simulink model "EPT"  (R2019b)
settings: Solver=FixedStepDiscrete  StartTime=0.0  StopTime=5  FixedStep=0.005  RelTol=1e-3  EnableMultiTasking=on
PreLoadFcn:
  | try, model_open; catch, disp('Error occurred while executing model pre-load callback: model_open.m'); disp('Please assure that the MATLAB working directory is set to the model directory before opening.'); end
InitFcn:
  | try, model_open; catch, end
undefined symbols (not defined in the file or in its folder): Bridge, GCM, H, ln, raptor_get_param_eval, raptor_get_safe_string, raptor_xcp_function
libraries: Raptor_lib x2810, simulink x374, hdlsllib x19
(part 12 of 45)

== system EPT/Foreground_TimeBase_5ms/CAN/CAN1_exec/BCU vs RMDA-BMS/BCU-OBU Status-OP G2 ==
  Trigger : TriggerPort  VariantControl=Variant  PortDimensions=1
  raptor_adjustment : Raptor_lib/Data Storage/raptor_adjustment  paramName='Cal_BP_OBU_AH_Def'  nameSource=Parameter  initValue=145  dataType=uint8  storage=Calibration  calDispType=Number  calEnum={'False', 'True'}  calGain=1.0  calOffset=0.0  calMax=inf  calMin=-inf  calFormat='-1'  calUnit=''  calHelp=''  calAccess=1  calFunction=raptor_xcp_function(gcb)  calDispHeaders=off  calColHeaders={'Col1' 'Col2' 'Col3'}  calRowHeaders={'Row1' 'Row2' 'Row3'}
      settings: SourceProductName=Raptor
  raptor_can_txmsg : Raptor_lib/CAN/raptor_can_txmsg  canDefinition=struct('dbcFile', 'BCU_OBU_HMI.dbc','message', 'BCU_OBU_Status_OP_G2','comment', '','signals', {{'BP_OBU_SOA','BP_OBU_SOC','BP_OBU_AH_Stored','BP_OBU_AH_FCC','BP_OBU_AH_Def'}},'enabled', [ 1 1 1 1 1;],'canBus', '''CAN1''','messageID', [ 1526;],'idMask', [ 536870911;],'payloadMask', [],'payloadValue', [],'period', [ 0;],'mailbox', '','queueSize', [ 1;],'label', [ 0;],'ver', [ 2;],'showID', [ 0;],'showRaw', [ 0;],'fill', [ 0;],'editID', [ 0;],'signalOrder', [ 2;])  canBus='CAN1'  queueSize=1  payloadMask=[]  payloadValue=[]  period=0  showID=0  label=0  idMask=hex2dec('1FFFFFFF')  fill=0  id=1526  showRaw=0  signalOrder=2  signalInfo={{struct('Name', 'BP_OBU_AH_Def','Startbit', [ 0;],'SignalSize', [ 8;],'ByteOrder', 'BigEndian','ValueType', 'UNSIGNED','Class', 'uint8','Signed', [ 0;],'Factor', [ 1;],'Offset', [ 0;],'Min', [ 0;],'Max', [ 0;],'Units', '','Comment', '','StartBit', [ 0;]),struct('Name', 'BP_OBU_AH_FCC','Startbit', [ 0;],'SignalSize', [ 8;],'ByteOrder', 'BigEndian','ValueType', 'UNSIGNED','Class', 'uint8','Signed', [ 0;],'Factor', [ 1;],'Offset', [ 0;],'Min', [ 0;],'Max', [ 0;],'Units', '','Comment', '','StartBit', [ 8;]),struct('Name', 'BP_OBU_AH_Stored','Startbit', [ 0;],'SignalSize', [ 8;],'ByteOrder', 'BigEndian','ValueType', 'UNSIGNED','Class', 'uint8','Signed', [ 0;],'Factor', [ 1;],'Offset', [ 0;],'Min', [ 0;],'Max', [ 0;],'Units', '','Comment', '','StartBit', [ 16;]),struct('Name', 'BP_OBU_SOC','Startbit', [ 0;],'SignalSize', [ 16;],'ByteOrder', 'BigEndian','ValueType', 'UNSIGNED','Class', 'uint16','Signed', [ 0;],'Factor', [ 0.1;],'Offset', [ -50;],'Min', [ 0;],'Max', [ 0;],'Units', '','Comment', '','StartBit', [ 32;]),struct('Name', 'BP_OBU_SOA','Startbit', [ 0;],'SignalSize', [ 8;],'ByteOrder', 'BigEndian','ValueType', 'UNSIGNED','Class', 'uint8','Signed', [ 0;],'Factor', [ 0.5;],'Offset', [ 0;],'Min', [ 0;],'Max', [ 0;],'Units', '','Comment', '','StartBit', [ 40;])}}
      settings: SourceProductName=Raptor
  raptor_data_def1 : Raptor_lib/Data Storage/raptor_data_def  dataName='EPT_BPOBU_FCCAP'  initValue=0  dataType=double  storage=Volatile (RAM)  calVisible=on  calType=Measurement  calDispType=Number  calEnum={'False', 'True'}  calGain=1.0  calOffset=0  calMin=-inf  calMax=inf  calFormat='-1'  calUnit=''  calHelp=''  calAccess=1  calFunction=raptor_xcp_function(gcb)  calDispHeaders=off  calColHeaders={'Col1' 'Col2' 'Col3'}  calRowHeaders={'Row1' 'Row2' 'Row3'}
      settings: SourceProductName=Raptor
  raptor_data_def2 : Raptor_lib/Data Storage/raptor_data_def  dataName='EPT_BPOBU_AH_Def'  initValue=0  dataType=uint8  storage=Volatile (RAM)  calVisible=on  calType=Measurement  calDispType=Number  calEnum={'False', 'True'}  calGain=1.0  calOffset=0  calMin=-inf  calMax=inf  calFormat='-1'  calUnit=''  calHelp=''  calAccess=1  calFunction=raptor_xcp_function(gcb)  calDispHeaders=off  calColHeaders={'Col1' 'Col2' 'Col3'}  calRowHeaders={'Row1' 'Row2' 'Row3'}
      settings: SourceProductName=Raptor
  raptor_data_def4 : Raptor_lib/Data Storage/raptor_data_def  dataName='BP_OBU_AH_Stored'  initValue=0  dataType=double  storage=Volatile (RAM)  calVisible=on  calType=Measurement  calDispType=Number  calEnum={'False', 'True'}  calGain=1.0  calOffset=0  calMin=-inf  calMax=inf  calFormat='-1'  calUnit=''  calHelp=''  calAccess=1  calFunction=raptor_xcp_function(gcb)  calDispHeaders=off  calColHeaders={'Col1' 'Col2' 'Col3'}  calRowHeaders={'Row1' 'Row2' 'Row3'}
      settings: SourceProductName=Raptor
  raptor_data_def5 : Raptor_lib/Data Storage/raptor_data_def  dataName='EPT_BPOBU_SOA'  initValue=0  dataType=double  storage=Volatile (RAM)  calVisible=on  calType=Measurement  calDispType=Number  calEnum={'False', 'True'}  calGain=1.0  calOffset=0  calMin=-inf  calMax=inf  calFormat='-1'  calUnit=''  calHelp=''  calAccess=1  calFunction=raptor_xcp_function(gcb)  calDispHeaders=off  calColHeaders={'Col1' 'Col2' 'Col3'}  calRowHeaders={'Row1' 'Row2' 'Row3'}
      settings: SourceProductName=Raptor
  raptor_data_read1 : Raptor_lib/Data Storage/raptor_data_read  dataName='EPT_BPOBU_SOC'  dataShape=Scalar  idxSource=Input  idxRow=1  idxCol=1
      settings: SourceProductName=Raptor
  raptor_data_read2 : Raptor_lib/Data Storage/raptor_data_read  dataName='BP_OBU_AH_Stored'  dataShape=Scalar  idxSource=Input  idxRow=1  idxCol=1
      settings: SourceProductName=Raptor
  raptor_data_read4 : Raptor_lib/Data Storage/raptor_data_read  dataName='EPT_BPOBU_FCCAP'  dataShape=Scalar  idxSource=Input  idxRow=1  idxCol=1
      settings: SourceProductName=Raptor
  raptor_data_read5 : Raptor_lib/Data Storage/raptor_data_read  dataName='EPT_BPOBU_AH_DEF'  dataShape=Scalar  idxSource=Input  idxRow=1  idxCol=1
      settings: SourceProductName=Raptor
  raptor_data_read7 : Raptor_lib/Data Storage/raptor_data_read  dataName='EPT_BPOBU_SOA'  dataShape=Scalar  idxSource=Input  idxRow=1  idxCol=1
      settings: SourceProductName=Raptor
  raptor_data_write : Raptor_lib/Data Storage/raptor_data_write  dataName='EPT_BPOBU_AH_DEF'  dataShape=Scalar  idxSource=Input Port  idxRow=1  idxCol=1
      settings: SourceProductName=Raptor
  wires:
  raptor_data_read5/1 -> raptor_can_txmsg/5
  raptor_data_read4/1 -> raptor_can_txmsg/4
  raptor_data_read1/1 -> raptor_can_txmsg/2
  raptor_data_read2/1 -> raptor_can_txmsg/3
  raptor_data_read7/1 -> raptor_can_txmsg/1
  raptor_adjustment/1 -> raptor_data_write/1

== system EPT/Foreground_TimeBase_5ms/CAN/CAN1_exec/BCU vs RMDA-BMS/BCU-OBU Status-OP G3 ==
  Trigger : TriggerPort  VariantControl=Variant  PortDimensions=1
  raptor_can_txmsg : Raptor_lib/CAN/raptor_can_txmsg  canDefinition=struct('dbcFile', 'BCU_OBU_HMI.dbc','message', 'BCU_OBU_Status_OP_G3','comment', '','signals', {{'NA_Cooling_CTL_OP','I2V_Batt_Volt','BP_OBU_Tair_in','BP_OBU_Tair_Out','BP_OBU_Tbp_Down','BP_OBU_Tbp_Up'}},'enabled', [ 1 1 1 1 1 1;],'canBus', '''CAN1''','messageID', [ 1527;],'idMask', [ 536870911;],'payloadMask', [],'payloadValue', [],'period', [ 0;],'mailbox', '','queueSize', [ 1;],'label', [ 0;],'ver', [ 2;],'showID', [ 0;],'showRaw', [ 0;],'fill', [ 0;],'editID', [ 0;],'signalOrder', [ 2;])  canBus='CAN1'  queueSize=1  payloadMask=[]  payloadValue=[]  period=0  showID=0  label=0  idMask=hex2dec('1FFFFFFF')  fill=0  id=1527  showRaw=0  signalOrder=2  signalInfo={{struct('Name', 'BP_OBU_Tbp_Up','Startbit', [ 0;],'SignalSize', [ 8;],'ByteOrder', 'BigEndian','ValueType', 'UNSIGNED','Class', 'uint8','Signed', [ 0;],'Factor', [ 0.5;],'Offset', [ -40;],'Min', [ 0;],'Max', [ 0;],'Units', '','Comment', '','StartBit', [ 0;]),struct('Name', 'BP_OBU_Tbp_Down','Startbit', [ 0;],'SignalSize', [ 8;],'ByteOrder', 'BigEndian','ValueType', 'UNSIGNED','Class', 'uint8','Signed', [ 0;],'Factor', [ 0.5;],'Offset', [ -40;],'Min', [ 0;],'Max', [ 0;],'Units', '','Comment', '','StartBit', [ 8;]),struct('Name', 'BP_OBU_Tair_Out','Startbit', [ 0;],'SignalSize', [ 8;],'ByteOrder', 'BigEndian','ValueType', 'UNSIGNED','Class', 'uint8','Signed', [ 0;],'Factor', [ 0.5;],'Offset', [ -40;],'Min', [ 0;],'Max', [ 0;],'Units', '','Comment', '','StartBit', [ 16;]),struct('Name', 'BP_OBU_Tair_in','Startbit', [ 0;],'SignalSize', [ 8;],'ByteOrder', 'BigEndian','ValueType', 'UNSIGNED','Class', 'uint8','Signed', [ 0;],'Factor', [ 0.5;],'Offset', [ -40;],'Min', [ 0;],'Max', [ 0;],'Units', '','Comment', '','StartBit', [ 24;]),struct('Name', 'I2V_Batt_Volt','Startbit', [ 0;],'SignalSize', [ 8;],'ByteOrder', 'BigEndian','ValueType', 'UNSIGNED','Class', 'uint8','Signed', [ 0;],'Factor', [ 0.1;],'Offset', [ 0;],'Min', [ 0;],'Max', [ 0;],'Units', '','Comment', '','StartBit', [ 32;]),struct('Name', 'NA_Cooling_CTL_OP','Startbit', [ 0;],'SignalSize', [ 8;],'ByteOrder', 'BigEndian','ValueType', 'UNSIGNED','Class', 'uint8','Signed', [ 0;],'Factor', [ 0.5;],'Offset', [ 0;],'Min', [ 0;],'Max', [ 0;],'Units', '','Comment', '','StartBit', [ 40;])}}
      settings: SourceProductName=Raptor
  raptor_data_def1 : Raptor_lib/Data Storage/raptor_data_def  dataName='BP_OBU_Tair_In'  initValue=0  dataType=double  storage=Volatile (RAM)  calVisible=on  calType=Measurement  calDispType=Number  calEnum={'False', 'True'}  calGain=1.0  calOffset=0  calMin=-inf  calMax=inf  calFormat='-1'  calUnit=''  calHelp=''  calAccess=1  calFunction=raptor_xcp_function(gcb)  calDispHeaders=off  calColHeaders={'Col1' 'Col2' 'Col3'}  calRowHeaders={'Row1' 'Row2' 'Row3'}
      settings: SourceProductName=Raptor
  raptor_data_def2 : Raptor_lib/Data Storage/raptor_data_def  dataName='BP_OBU_Tair_Out'  initValue=0  dataType=double  storage=Volatile (RAM)  calVisible=on  calType=Measurement  calDispType=Number  calEnum={'False', 'True'}  calGain=1.0  calOffset=0  calMin=-inf  calMax=inf  calFormat='-1'  calUnit=''  calHelp=''  calAccess=1  calFunction=raptor_xcp_function(gcb)  calDispHeaders=off  calColHeaders={'Col1' 'Col2' 'Col3'}  calRowHeaders={'Row1' 'Row2' 'Row3'}
      settings: SourceProductName=Raptor
  raptor_data_read1 : Raptor_lib/Data Storage/raptor_data_read  dataName='I2V_Battery_Volt'  dataShape=Scalar  idxSource=Input  idxRow=1  idxCol=1
      settings: SourceProductName=Raptor
  raptor_data_read3 : Raptor_lib/Data Storage/raptor_data_read  dataName='BP_OBU_Tair_In'  dataShape=Scalar  idxSource=Input  idxRow=1  idxCol=1
      settings: SourceProductName=Raptor
  raptor_data_read4 : Raptor_lib/Data Storage/raptor_data_read  dataName='BP_OBU_Tair_Out'  dataShape=Scalar  idxSource=Input  idxRow=1  idxCol=1
      settings: SourceProductName=Raptor
  raptor_data_read5 : Raptor_lib/Data Storage/raptor_data_read  dataName='BP_OBU_Tbp_Down'  dataShape=Scalar  idxSource=Input  idxRow=1  idxCol=1
      settings: SourceProductName=Raptor
  raptor_data_read6 : Raptor_lib/Data Storage/raptor_data_read  dataName='BP_OBU_Tbp_Up'  dataShape=Scalar  idxSource=Input  idxRow=1  idxCol=1
      settings: SourceProductName=Raptor
  wires:
  raptor_data_read1/1 -> raptor_can_txmsg/2
  raptor_data_read4/1 -> raptor_can_txmsg/4
  raptor_data_read5/1 -> raptor_can_txmsg/5
  raptor_data_read6/1 -> raptor_can_txmsg/6
  raptor_data_read3/1 -> raptor_can_txmsg/3

== system EPT/Foreground_TimeBase_5ms/CAN/CAN1_exec/BCU vs RMDA-BMS/BCU-OBU Status-OP G4  ==
  Trigger : TriggerPort  VariantControl=Variant  PortDimensions=1
  raptor_can_txmsg : Raptor_lib/CAN/raptor_can_txmsg  canDefinition=struct('dbcFile', 'BCU_OBU_HMI.dbc','message', 'BCU_OBU_Status_OP_G4','comment', '','signals', {{'Min_CellT','Max_CellT','Min_CellV','Max_CellV'}},'enabled', [ 1 1 1 1;],'canBus', '''CAN1''','messageID', [ 1528;],'idMask', [ 536870911;],'payloadMask', [],'payloadValue', [],'period', [ 0;],'mailbox', '','queueSize', [ 1;],'label', [ 0;],'ver', [ 2;],'showID', [ 0;],'showRaw', [ 0;],'fill', [ 0;],'editID', [ 0;],'signalOrder', [ 2;])  canBus='CAN1'  queueSize=1  payloadMask=[]  payloadValue=[]  period=0  showID=0  label=0  idMask=hex2dec('1FFFFFFF')  fill=0  id=1528  showRaw=0  signalOrder=2  signalInfo={{struct('Name', 'Max_CellV','Startbit', [ 0;],'SignalSize', [ 16;],'ByteOrder', 'BigEndian','ValueType', 'UNSIGNED','Class', 'uint16','Signed', [ 0;],'Factor', [ 0.001;],'Offset', [ 0;],'Min', [ 0;],'Max', [ 0;],'Units', '','Comment', '','StartBit', [ 8;]),struct('Name', 'Min_CellV','Startbit', [ 0;],'SignalSize', [ 16;],'ByteOrder', 'BigEndian','ValueType', 'UNSIGNED','Class', 'uint16','Signed', [ 0;],'Factor', [ 0.001;],'Offset', [ 0;],'Min', [ 0;],'Max', [ 0;],'Units', '','Comment', '','StartBit', [ 24;]),struct('Name', 'Max_CellT','Startbit', [ 0;],'SignalSize', [ 8;],'ByteOrder', 'BigEndian','ValueType', 'UNSIGNED','Class', 'uint8','Signed', [ 0;],'Factor', [ 0.5;],'Offset', [ -40;],'Min', [ 0;],'Max', [ 0;],'Units', '','Comment', '','StartBit', [ 32;]),struct('Name', 'Min_CellT','Startbit', [ 0;],'SignalSize', [ 8;],'ByteOrder', 'BigEndian','ValueType', 'UNSIGNED','Class', 'uint8','Signed', [ 0;],'Factor', [ 0.5;],'Offset', [ -40;],'Min', [ 0;],'Max', [ 0;],'Units', '','Comment', '','StartBit', [ 40;])}}
      settings: SourceProductName=Raptor
  raptor_data_read1 : Raptor_lib/Data Storage/raptor_data_read  dataName='Max_CellT'  dataShape=Scalar  idxSource=Input  idxRow=1  idxCol=1
      settings: SourceProductName=Raptor
  raptor_data_read2 : Raptor_lib/Data Storage/raptor_data_read  dataName='Min_CellT'  dataShape=Scalar  idxSource=Input  idxRow=1  idxCol=1
      settings: SourceProductName=Raptor
  raptor_data_read4 : Raptor_lib/Data Storage/raptor_data_read  dataName='Max_CellV'  dataShape=Scalar  idxSource=Input  idxRow=1  idxCol=1
      settings: SourceProductName=Raptor
  raptor_data_read5 : Raptor_lib/Data Storage/raptor_data_read  dataName='Min_CellV'  dataShape=Scalar  idxSource=Input  idxRow=1  idxCol=1
      settings: SourceProductName=Raptor
  wires:
  raptor_data_read5/1 -> raptor_can_txmsg/3
  raptor_data_read4/1 -> raptor_can_txmsg/4
  raptor_data_read1/1 -> raptor_can_txmsg/2
  raptor_data_read2/1 -> raptor_can_txmsg/1

== system EPT/Foreground_TimeBase_5ms/CAN/CAN1_exec/BCU vs RMDA-BMS/BP-OBU Enable CTL & OP Status  ==
  Trigger : TriggerPort  VariantControl=Variant  PortDimensions=1
  BP-OBU Enable CTL : Subsystem
  BP-OBU Output Mode : Subsystem
  BP-OBU_Enable Mode : Subsystem
  BP-OBU_HV CTL Mode : Subsystem
  BP-OBU_OP Mode : Subsystem
  EPT Status Bitmap : Subsystem
  raptor_can_txmsg : Raptor_lib/CAN/raptor_can_txmsg  canDefinition=struct('dbcFile', 'BCU_OBU_HMI.dbc','message', 'BP_OBU_Enable_CTLandOP_Status','comment', '','signals', {{'BP_OBU_HV_CTL_Mode','BP_OBU_Enable_Mode','BP_OBU_OP_Mode','BP_OBU_Output_Mode','BP_OBU_Enable_CTL','EPT_Status_Bitmap'}},'enabled', [ 1 1 1 1 1 1;],'canBus', '''CAN1''','messageID', [ 1523;],'idMask', [ 536870911;],'payloadMask', [],'payloadValue', [],'period', [ 0;],'mailbox', '','queueSize', [ 1;],'label', [ 0;],'ver', [ 2;],'showID', [ 0;],'showRaw', [ 0;],'fill', [ 0;],'editID', [ 0;],'signalOrder', [ 2;])  canBus='CAN1'  queueSize=1  payloadMask=[]  payloadValue=[]  period=0  showID=0  label=0  idMask=hex2dec('1FFFFFFF')  fill=0  id=1523  showRaw=0  signalOrder=2  signalInfo={{struct('Name', 'EPT_Status_Bitmap','Startbit', [ 0;],'SignalSize', [ 8;],'ByteOrder', 'BigEndian','ValueType', 'UNSIGNED','Class', 'uint8','Signed', [ 0;],'Factor', [ 1;],'Offset', [ 0;],'Min', [ 0;],'Max', [ 0;],'Units', '','Comment', '','StartBit', [ 0;]),struct('Name', 'BP_OBU_Output_Mode','Startbit', [ 0;],'SignalSize', [ 8;],'ByteOrder', 'BigEndian','ValueType', 'UNSIGNED','Class', 'uint8','Signed', [ 0;],'Factor', [ 1;],'Offset', [ 0;],'Min', [ 0;],'Max', [ 0;],'Units', '','Comment', '','StartBit', [ 16;]),struct('Name', 'BP_OBU_OP_Mode','Startbit', [ 0;],'SignalSize', [ 8;],'ByteOrder', 'BigEndian','ValueType', 'UNSIGNED','Class', 'uint8','Signed', [ 0;],'Factor', [ 1;],'Offset', [ 0;],'Min', [ 0;],'Max', [ 0;],'Units', '','Comment', '','StartBit', [ 32;]),struct('Name', 'BP_OBU_HV_CTL_Mode','Startbit', [ 0;],'SignalSize', [ 8;],'ByteOrder', 'BigEndian','ValueType', 'UNSIGNED','Class', 'uint8','Signed', [ 0;],'Factor', [ 1;],'Offset', [ 0;],'Min', [ 0;],'Max', [ 0;],'Units', '','Comment', '','StartBit', [ 48;]),struct('Name', 'BP_OBU_Enable_Mode','Startbit', [ 0;],'SignalSize', [ 8;],'ByteOrder', 'BigEndian','ValueType', 'UNSIGNED','Class', 'uint8','Signed', [ 0;],'Factor', [ 1;],'Offset', [ 0;],'Min', [ 0;],'Max', [ 0;],'Units', '','Comment', '','StartBit', [ 40;]),struct('Name', 'BP_OBU_Enable_CTL','Startbit', [ 0;],'SignalSize', [ 8;],'ByteOrder', 'BigEndian','ValueType', 'UNSIGNED','Class', 'uint8','Signed', [ 0;],'Factor', [ 1;],'Offset', [ 0;],'Min', [ 0;],'Max', [ 0;],'Units', '','Comment', '','StartBit', [ 8;])}}
      settings: SourceProductName=Raptor
  wires:
  BP-OBU_HV CTL Mode/1(BP-OBU_HV CTL Mode) -> raptor_can_txmsg/1
  BP-OBU_Enable Mode/1(BP-OBU_Enable Mode) -> raptor_can_txmsg/2
  BP-OBU Output Mode/1(BP-OBU Output Mode) -> raptor_can_txmsg/4
  EPT Status Bitmap/1(EPT Status Bitmap) -> raptor_can_txmsg/6
  BP-OBU Enable CTL/1(BP-OBU Enable CTL) -> raptor_can_txmsg/5
  BP-OBU_OP Mode/1(BP-OBU_OP Mode) -> raptor_can_txmsg/3

== system EPT/Foreground_TimeBase_5ms/CAN/CAN1_exec/BCU vs RMDA-BMS/Remote DAG2-5E0 ==
  Trigger : TriggerPort  VariantControl=Variant  PortDimensions=1
  Bitwise Operator : simulink/Logic and Bit Operations/Bitwise Operator  logicop=AND  UseBitMask=on  BitMask=hex2dec('f0')  BitMaskRealWorld=Stored Integer
  Bitwise Operator1 : simulink/Logic and Bit Operations/Bitwise Operator  logicop=AND  UseBitMask=on  BitMask=hex2dec('0f')  BitMaskRealWorld=Stored Integer
  Data Type Conversion{,1..5} (6 alike) : DataTypeConversion
  Fcn3 : Fcn  Expr=(u(1)+12.5)/0.5
  Shift Arithmetic1 : ArithShift  BitShiftNumber=4  BitShiftDirection=Right
  raptor_can_txmsg : Raptor_lib/CAN/raptor_can_txmsg  canDefinition=struct('dbcFile', 'BCUvsRMDA_CMU.dbc','message', 'RemoteDAG_5E0','comment', '','signals', {{'CMU1_EW_Level3_Hbyte','CMU1_EW_Level3_Lbyte','CMU1_FCC','CMU1_Mode','CMU1_RCAP','CMU1_RSOC'}},'enabled', [ 1 1 1 1 1 1;],'canBus', '''CAN1''','messageID', [ 1504;],'idMask', [ 536870911;],'payloadMask', [],'payloadValue', [],'period', [ 0;],'mailbox', '','queueSize', [ 1;],'label', [ 0;],'ver', [ 2;],'showID', [ 0;],'showRaw', [ 0;],'fill', [ 0;],'editID', [ 0;],'signalOrder', [ 1;])  canBus='CAN1'  queueSize=1  payloadMask=[]  payloadValue=[]  period=0  showID=0  label=0  idMask=hex2dec('1FFFFFFF')  fill=0  id=1504  showRaw=0  signalOrder=1  signalInfo={{struct('Name', 'CMU1_Mode','Startbit', [ 0;],'SignalSize', [ 8;],'ByteOrder', 'BigEndian','ValueType', 'UNSIGNED','Class', 'uint8','Signed', [ 0;],'Factor', [ 1;],'Offset', [ 0;],'Min', [ 0;],'Max', [ 0;],'Units', '','Comment', '','StartBit', [ 0;]),struct('Name', 'CMU1_EW_Level3_Hbyte','Startbit', [ 0;],'SignalSize', [ 8;],'ByteOrder', 'BigEndian','ValueType', 'UNSIGNED','Class', 'uint8','Signed', [ 0;],'Factor', [ 1;],'Offset', [ 0;],'Min', [ 0;],'Max', [ 0;],'Units', '','Comment', '','StartBit', [ 8;]),struct('Name', 'CMU1_EW_Level3_Lbyte','Startbit', [ 0;],'SignalSize', [ 8;],'ByteOrder', 'BigEndian','ValueType', 'UNSIGNED','Class', 'uint8','Signed', [ 0;],'Factor', [ 1;],'Offset', [ 0;],'Min', [ 0;],'Max', [ 0;],'Units', '','Comment', '','StartBit', [ 16;]),struct('Name', 'CMU1_FCC','Startbit', [ 0;],'SignalSize', [ 8;],'ByteOrder', 'BigEndian','ValueType', 'UNSIGNED','Class', 'uint8','Signed', [ 0;],'Factor', [ 1;],'Offset', [ 0;],'Min', [ 0;],'Max', [ 0;],'Units', '','Comment', '','StartBit', [ 32;]),struct('Name', 'CMU1_RCAP','Startbit', [ 0;],'SignalSize', [ 8;],'ByteOrder', 'BigEndian','ValueType', 'UNSIGNED','Class', 'uint8','Signed', [ 0;],'Factor', [ 1;],'Offset', [ 0;],'Min', [ 0;],'Max', [ 0;],'Units', '','Comment', '','StartBit', [ 40;]),struct('Name', 'CMU1_RSOC','Startbit', [ 0;],'SignalSize', [ 8;],'ByteOrder', 'BigEndian','ValueType', 'UNSIGNED','Class', 'uint8','Signed', [ 0;],'Factor', [ 1;],'Offset', [ 0;],'Min', [ 0;],'Max', [ 0;],'Units', '','Comment', '','StartBit', [ 48;])}}
      settings: SourceProductName=Raptor
  raptor_data_read2 : Raptor_lib/Data Storage/raptor_data_read  dataName='Rx_0x200B2A1_FCC'  dataShape=Scalar  idxSource=Input  idxRow=1  idxCol=1
      settings: SourceProductName=Raptor
  raptor_data_read3 : Raptor_lib/Data Storage/raptor_data_read  dataName='Rx_0x200B0A1_CMU1_Status'  dataShape=Scalar  idxSource=Input  idxRow=1  idxCol=1
      settings: SourceProductName=Raptor
  raptor_data_read4 : Raptor_lib/Data Storage/raptor_data_read  dataName='Rx_0x200B2A1_RC'  dataShape=Scalar  idxSource=Input  idxRow=1  idxCol=1
      settings: SourceProductName=Raptor
  raptor_data_read5 : Raptor_lib/Data Storage/raptor_data_read  dataName='Rx_0x200B2A1_RSOC'  dataShape=Scalar  idxSource=Input  idxRow=1  idxCol=1
      settings: SourceProductName=Raptor
  raptor_data_read6 : Raptor_lib/Data Storage/raptor_data_read  dataName='Rx_0x200BAA1_Event3_Error_Code'  dataShape=Scalar  idxSource=Input  idxRow=1  idxCol=1
      settings: SourceProductName=Raptor
  wires:
  raptor_data_read2/1 -> Data Type Conversion5/1
  raptor_data_read4/1 -> Data Type Conversion4/1
  raptor_data_read5/1 -> Fcn3/1
  raptor_data_read6/1 -> Bitwise Operator/1, Bitwise Operator1/1
  Bitwise Operator/1 -> Shift Arithmetic1/1
  Bitwise Operator1/1 -> Data Type Conversion/1
  Shift Arithmetic1/1 -> Data Type Conversion1/1
  Data Type Conversion1/1 -> raptor_can_txmsg/1
  Data Type Conversion2/1 -> raptor_can_txmsg/2
  Data Type Conversion/1 -> Data Type Conversion2/1
  Data Type Conversion5/1 -> raptor_can_txmsg/3
  raptor_data_read3/1 -> raptor_can_txmsg/4
  Fcn3/1 -> Data Type Conversion3/1
  Data Type Conversion3/1 -> raptor_can_txmsg/6
  Data Type Conversion4/1 -> raptor_can_txmsg/5

== system EPT/Foreground_TimeBase_5ms/CAN/CAN1_exec/BCU vs RMDA-BMS/Remote DAG2-5E1 ==
  Trigger : TriggerPort  VariantControl=Variant  PortDimensions=1
  Data Type Conversion{1..4} (4 alike) : DataTypeConversion
  Fcn1 : Fcn  Expr=(u(1)-2)/0.01
  Fcn2 : Fcn  Expr=(u(1)-2)/0.01
  Fcn3 : Fcn  Expr=(u(1)+40)/0.5
  Fcn4 : Fcn  Expr=(u(1)+40)/0.5
  raptor_can_txmsg : Raptor_lib/CAN/raptor_can_txmsg  canDefinition=struct('dbcFile', 'BCUvsRMDA_CMU.dbc','message', 'RemoteDAG_5E1','comment', '','signals', {{'CMU1_Ibp','CMU1_Tcell_Max','CMU1_Tcell_Min','CMU1_Vbp','CMU1_Vcell_Max','CMU1_Vcell_Min'}},'enabled', [ 1 1 1 1 1 1;],'canBus', '''CAN1''','messageID', [ 1505;],'idMask', [ 536870911;],'payloadMask', [],'payloadValue', [],'period', [ 0;],'mailbox', '','queueSize', [ 1;],'label', [ 0;],'ver', [ 2;],'showID', [ 0;],'showRaw', [ 0;],'fill', [ 0;],'editID', [ 0;],'signalOrder', [ 1;])  canBus='CAN1'  queueSize=1  payloadMask=[]  payloadValue=[]  period=0  showID=0  label=0  idMask=hex2dec('1FFFFFFF')  fill=0  id=1505  showRaw=0  signalOrder=1  signalInfo={{struct('Name', 'CMU1_Ibp','Startbit', [ 0;],'SignalSize', [ 16;],'ByteOrder', 'BigEndian','ValueType', 'UNSIGNED','Class', 'uint16','Signed', [ 0;],'Factor', [ 0.02;],'Offset', [ -500;],'Min', [ 0;],'Max', [ 0;],'Units', '','Comment', '','StartBit', [ 8;]),struct('Name', 'CMU1_Vbp','Startbit', [ 0;],'SignalSize', [ 16;],'ByteOrder', 'BigEndian','ValueType', 'UNSIGNED','Class', 'uint16','Signed', [ 0;],'Factor', [ 0.01;],'Offset', [ 0;],'Min', [ 0;],'Max', [ 0;],'Units', '','Comment', '','StartBit', [ 24;]),struct('Name', 'CMU1_Vcell_Max','Startbit', [ 0;],'SignalSize', [ 8;],'ByteOrder', 'BigEndian','ValueType', 'UNSIGNED','Class', 'uint8','Signed', [ 0;],'Factor', [ 1;],'Offset', [ 0;],'Min', [ 0;],'Max', [ 0;],'Units', '','Comment', '','StartBit', [ 32;]),struct('Name', 'CMU1_Vcell_Min','Startbit', [ 0;],'SignalSize', [ 8;],'ByteOrder', 'BigEndian','ValueType', 'UNSIGNED','Class', 'uint8','Signed', [ 0;],'Factor', [ 1;],'Offset', [ 0;],'Min', [ 0;],'Max', [ 0;],'Units', '','Comment', '','StartBit', [ 40;]),struct('Name', 'CMU1_Tcell_Max','Startbit', [ 0;],'SignalSize', [ 8;],'ByteOrder', 'BigEndian','ValueType', 'UNSIGNED','Class', 'uint8','Signed', [ 0;],'Factor', [ 1;],'Offset', [ 0;],'Min', [ 0;],'Max', [ 0;],'Units', '','Comment', '','StartBit', [ 48;]),struct('Name', 'CMU1_Tcell_Min','Startbit', [ 0;],'SignalSize', [ 8;],'ByteOrder', 'BigEndian','ValueType', 'UNSIGNED','Class', 'uint8','Signed', [ 0;],'Factor', [ 1;],'Offset', [ 0;],'Min', [ 0;],'Max', [ 0;],'Units', '','Comment', '','StartBit', [ 56;])}}
      settings: SourceProductName=Raptor
  raptor_data_read : Raptor_lib/Data Storage/raptor_data_read  dataName='Rx_0x200B0A1_Max_Cell_Volt'  dataShape=Scalar  idxSource=Input  idxRow=1  idxCol=1
      settings: SourceProductName=Raptor
  raptor_data_read1 : Raptor_lib/Data Storage/raptor_data_read  dataName='Rx_0x200B0A1_Min_Cell_Volt'  dataShape=Scalar  idxSource=Input  idxRow=1  idxCol=1
      settings: SourceProductName=Raptor
  raptor_data_read2 : Raptor_lib/Data Storage/raptor_data_read  dataName='Rx_0x200B1A1_Min_Cell_Temp'  dataShape=Scalar  idxSource=Input  idxRow=1  idxCol=1
      settings: SourceProductName=Raptor
  raptor_data_read3 : Raptor_lib/Data Storage/raptor_data_read  dataName='Rx_0x200B0A1_Battery_Current'  dataShape=Scalar  idxSource=Input  idxRow=1  idxCol=1
      settings: SourceProductName=Raptor
  raptor_data_read4 : Raptor_lib/Data Storage/raptor_data_read  dataName='Rx_0x200B1A1_BatteryVolt'  dataShape=Scalar  idxSource=Input  idxRow=1  idxCol=1
      settings: SourceProductName=Raptor
  raptor_data_read5 : Raptor_lib/Data Storage/raptor_data_read  dataName='Rx_0x200B1A1_Max_Cell_Temp'  dataShape=Scalar  idxSource=Input  idxRow=1  idxCol=1
      settings: SourceProductName=Raptor
  wires:
  raptor_data_read/1 -> Fcn2/1
  raptor_data_read1/1 -> Fcn1/1
  raptor_data_read3/1 -> raptor_can_txmsg/1
  raptor_data_read4/1 -> raptor_can_txmsg/4
  Fcn2/1 -> Data Type Conversion1/1
  Fcn1/1 -> Data Type Conversion4/1
  Data Type Conversion4/1 -> raptor_can_txmsg/6
  Data Type Conversion1/1 -> raptor_can_txmsg/5
  Fcn3/1 -> Data Type Conversion2/1
  Data Type Conversion2/1 -> raptor_can_txmsg/2
  raptor_data_read5/1 -> Fcn3/1
  raptor_data_read2/1 -> Fcn4/1
  Data Type Conversion3/1 -> raptor_can_txmsg/3
  Fcn4/1 -> Data Type Conversion3/1

== system EPT/Foreground_TimeBase_5ms/CAN/CAN1_exec/BCU vs RMDA-BMS/Remote DAG2-5E2 ==
  Trigger : TriggerPort  VariantControl=Variant  PortDimensions=1
  Data Type Conversion{1..8} (8 alike) : DataTypeConversion
  Fcn{,1..7} (8 alike) : Fcn  Expr=(u(1)-2)/0.01
  raptor_can_txmsg : Raptor_lib/CAN/raptor_can_txmsg  canDefinition=struct('dbcFile', 'BCUvsRMDA_CMU.dbc','message', 'RemoteDAG_5E2','comment', '','signals', {{'CMU1_Vcell_V01','CMU1_Vcell_V02','CMU1_Vcell_V03','CMU1_Vcell_V04','CMU1_Vcell_V05','CMU1_Vcell_V06','CMU1_Vcell_V07','CMU1_Vcell_V08'}},'enabled', [ 1 1 1 1 1 1 1 1;],'canBus', '''CAN1''','messageID', [ 1506;],'idMask', [ 536870911;],'payloadMask', [],'payloadValue', [],'period', [ 0;],'mailbox', '','queueSize', [ 1;],'label', [ 0;],'ver', [ 2;],'showID', [ 0;],'showRaw', [ 0;],'fill', [ 0;],'editID', [ 0;],'signalOrder', [ 1;])  canBus='CAN1'  queueSize=1  payloadMask=[]  payloadValue=[]  period=0  showID=0  label=0  idMask=hex2dec('1FFFFFFF')  fill=0  id=1506  showRaw=0  signalOrder=1  signalInfo={{struct('Name', 'CMU1_Vcell_V01','Startbit', [ 0;],'SignalSize', [ 8;],'ByteOrder', 'BigEndian','ValueType', 'UNSIGNED','Class', 'uint8','Signed', [ 0;],'Factor', [ 1;],'Offset', [ 0;],'Min', [ 0;],'Max', [ 0;],'Units', '','Comment', '','StartBit', [ 0;]),struct('Name', 'CMU1_Vcell_V02','Startbit', [ 0;],'SignalSize', [ 8;],'ByteOrder', 'BigEndian','ValueType', 'UNSIGNED','Class', 'uint8','Signed', [ 0;],'Factor', [ 1;],'Offset', [ 0;],'Min', [ 0;],'Max', [ 0;],'Units', '','Comment', '','StartBit', [ 8;]),struct('Name', 'CMU1_Vcell_V03','Startbit', [ 0;],'SignalSize', [ 8;],'ByteOrder', 'BigEndian','ValueType', 'UNSIGNED','Class', 'uint8','Signed', [ 0;],'Factor', [ 1;],'Offset', [ 0;],'Min', [ 0;],'Max', [ 0;],'Units', '','Comment', '','StartBit', [ 16;]),struct('Name', 'CMU1_Vcell_V04','Startbit', [ 0;],'SignalSize', [ 8;],'ByteOrder', 'BigEndian','ValueType', 'UNSIGNED','Class', 'uint8','Signed', [ 0;],'Factor', [ 1;],'Offset', [ 0;],'Min', [ 0;],'Max', [ 0;],'Units', '','Comment', '','StartBit', [ 24;]),struct('Name', 'CMU1_Vcell_V05','Startbit', [ 0;],'SignalSize', [ 8;],'ByteOrder', 'BigEndian','ValueType', 'UNSIGNED','Class', 'uint8','Signed', [ 0;],'Factor', [ 1;],'Offset', [ 0;],'Min', [ 0;],'Max', [ 0;],'Units', '','Comment', '','StartBit', [ 32;]),struct('Name', 'CMU1_Vcell_V06','Startbit', [ 0;],'SignalSize', [ 8;],'ByteOrder', 'BigEndian','ValueType', 'UNSIGNED','Class', 'uint8','Signed', [ 0;],'Factor', [ 1;],'Offset', [ 0;],'Min', [ 0;],'Max', [ 0;],'Units', '','Comment', '','StartBit', [ 40;]),struct('Name', 'CMU1_Vcell_V07','Startbit', [ 0;],'SignalSize', [ 8;],'ByteOrder', 'BigEndian','ValueType', 'UNSIGNED','Class', 'uint8','Signed', [ 0;],'Factor', [ 1;],'Offset', [ 0;],'Min', [ 0;],'Max', [ 0;],'Units', '','Comment', '','StartBit', [ 48;]),struct('Name', 'CMU1_Vcell_V08','Startbit', [ 0;],'SignalSize', [ 8;],'ByteOrder', 'BigEndian','ValueType', 'UNSIGNED','Class', 'uint8','Signed', [ 0;],'Factor', [ 1;],'Offset', [ 0;],'Min', [ 0;],'Max', [ 0;],'Units', '','Comment', '','StartBit', [ 56;])}}
      settings: SourceProductName=Raptor
  raptor_data_read : Raptor_lib/Data Storage/raptor_data_read  dataName='Rx_0x200C0A1_Cell_1_Volt'  dataShape=Scalar  idxSource=Input  idxRow=1  idxCol=1
      settings: SourceProductName=Raptor
  raptor_data_read1 : Raptor_lib/Data Storage/raptor_data_read  dataName='Rx_0x200C0A1_Cell_2_Volt'  dataShape=Scalar  idxSource=Input  idxRow=1  idxCol=1
      settings: SourceProductName=Raptor
  raptor_data_read2 : Raptor_lib/Data Storage/raptor_data_read  dataName='Rx_0x200C0A1_Cell_3_Volt'  dataShape=Scalar  idxSource=Input  idxRow=1  idxCol=1
      settings: SourceProductName=Raptor
  raptor_data_read3 : Raptor_lib/Data Storage/raptor_data_read  dataName='Rx_0x200C0A1_Cell_4_Volt'  dataShape=Scalar  idxSource=Input  idxRow=1  idxCol=1
      settings: SourceProductName=Raptor
  raptor_data_read4 : Raptor_lib/Data Storage/raptor_data_read  dataName='Rx_0x200C1A1_Cell_5_Volt'  dataShape=Scalar  idxSource=Input  idxRow=1  idxCol=1
      settings: SourceProductName=Raptor
  raptor_data_read5 : Raptor_lib/Data Storage/raptor_data_read  dataName='Rx_0x200C1A1_Cell_6_Volt'  dataShape=Scalar  idxSource=Input  idxRow=1  idxCol=1
      settings: SourceProductName=Raptor
  raptor_data_read6 : Raptor_lib/Data Storage/raptor_data_read  dataName='Rx_0x200C1A1_Cell_7_Volt'  dataShape=Scalar  idxSource=Input  idxRow=1  idxCol=1
      settings: SourceProductName=Raptor
  raptor_data_read7 : Raptor_lib/Data Storage/raptor_data_read  dataName='Rx_0x200C1A1_Cell_8_Volt'  dataShape=Scalar  idxSource=Input  idxRow=1  idxCol=1
      settings: SourceProductName=Raptor
  wires:
  raptor_data_read1/1 -> Fcn1/1
  raptor_data_read7/1 -> Fcn7/1
  Fcn5/1 -> Data Type Conversion1/1
  Fcn/1 -> Data Type Conversion4/1
  Fcn6/1 -> Data Type Conversion2/1
  Fcn4/1 -> Data Type Conversion5/1
  Fcn3/1 -> Data Type Conversion6/1
  Data Type Conversion3/1 -> raptor_can_txmsg/8
  Data Type Conversion7/1 -> raptor_can_txmsg/3
  Data Type Conversion6/1 -> raptor_can_txmsg/4
  Data Type Conversion5/1 -> raptor_can_txmsg/5
  Data Type Conversion1/1 -> raptor_can_txmsg/6
  Data Type Conversion8/1 -> raptor_can_txmsg/2
  Data Type Conversion2/1 -> raptor_can_txmsg/7
  Fcn7/1 -> Data Type Conversion3/1
  Fcn2/1 -> Data Type Conversion7/1
  Fcn1/1 -> Data Type Conversion8/1
  Data Type Conversion4/1 -> raptor_can_txmsg/1
  raptor_data_read/1 -> Fcn/1
  raptor_data_read2/1 -> Fcn2/1
  raptor_data_read3/1 -> Fcn3/1
  raptor_data_read4/1 -> Fcn4/1
  raptor_data_read5/1 -> Fcn5/1
  raptor_data_read6/1 -> Fcn6/1

== system EPT/Foreground_TimeBase_5ms/CAN/CAN1_exec/BCU vs RMDA-BMS/Remote DAG2-5E3 ==
  Trigger : TriggerPort  VariantControl=Variant  PortDimensions=1
  Data Type Conversion{1..8} (8 alike) : DataTypeConversion
  Fcn{,1..7} (8 alike) : Fcn  Expr=(u(1)-2)/0.01
  raptor_can_txmsg : Raptor_lib/CAN/raptor_can_txmsg  canDefinition=struct('dbcFile', 'BCUvsRMDA_CMU.dbc','message', 'RemoteDAG_5E3','comment', '','signals', {{'CMU1_Vcell_V09','CMU1_Vcell_V10','CMU1_Vcell_V11','CMU1_Vcell_V12','CMU1_Vcell_V13','CMU1_Vcell_V14','CMU1_Vcell_V15','CMU1_Vcell_V16'}},'enabled', [ 1 1 1 1 1 1 1 1;],'canBus', '''CAN1''','messageID', [ 1507;],'idMask', [ 536870911;],'payloadMask', [],'payloadValue', [],'period', [ 0;],'mailbox', '','queueSize', [ 1;],'label', [ 0;],'ver', [ 2;],'showID', [ 0;],'showRaw', [ 0;],'fill', [ 0;],'editID', [ 0;],'signalOrder', [ 1;])  canBus='CAN1'  queueSize=1  payloadMask=[]  payloadValue=[]  period=0  showID=0  label=0  idMask=hex2dec('1FFFFFFF')  fill=0  id=1507  showRaw=0  signalOrder=1  signalInfo={{struct('Name', 'CMU1_Vcell_V09','Startbit', [ 0;],'SignalSize', [ 8;],'ByteOrder', 'BigEndian','ValueType', 'UNSIGNED','Class', 'uint8','Signed', [ 0;],'Factor', [ 1;],'Offset', [ 0;],'Min', [ 0;],'Max', [ 0;],'Units', '','Comment', '','StartBit', [ 0;]),struct('Name', 'CMU1_Vcell_V10','Startbit', [ 0;],'SignalSize', [ 8;],'ByteOrder', 'BigEndian','ValueType', 'UNSIGNED','Class', 'uint8','Signed', [ 0;],'Factor', [ 1;],'Offset', [ 0;],'Min', [ 0;],'Max', [ 0;],'Units', '','Comment', '','StartBit', [ 8;]),struct('Name', 'CMU1_Vcell_V11','Startbit', [ 0;],'SignalSize', [ 8;],'ByteOrder', 'BigEndian','ValueType', 'UNSIGNED','Class', 'uint8','Signed', [ 0;],'Factor', [ 1;],'Offset', [ 0;],'Min', [ 0;],'Max', [ 0;],'Units', '','Comment', '','StartBit', [ 16;]),struct('Name', 'CMU1_Vcell_V12','Startbit', [ 0;],'SignalSize', [ 8;],'ByteOrder', 'BigEndian','ValueType', 'UNSIGNED','Class', 'uint8','Signed', [ 0;],'Factor', [ 1;],'Offset', [ 0;],'Min', [ 0;],'Max', [ 0;],'Units', '','Comment', '','StartBit', [ 24;]),struct('Name', 'CMU1_Vcell_V13','Startbit', [ 0;],'SignalSize', [ 8;],'ByteOrder', 'BigEndian','ValueType', 'UNSIGNED','Class', 'uint8','Signed', [ 0;],'Factor', [ 1;],'Offset', [ 0;],'Min', [ 0;],'Max', [ 0;],'Units', '','Comment', '','StartBit', [ 32;]),struct('Name', 'CMU1_Vcell_V14','Startbit', [ 0;],'SignalSize', [ 8;],'ByteOrder', 'BigEndian','ValueType', 'UNSIGNED','Class', 'uint8','Signed', [ 0;],'Factor', [ 1;],'Offset', [ 0;],'Min', [ 0;],'Max', [ 0;],'Units', '','Comment', '','StartBit', [ 40;]),struct('Name', 'CMU1_Vcell_V15','Startbit', [ 0;],'SignalSize', [ 8;],'ByteOrder', 'BigEndian','ValueType', 'UNSIGNED','Class', 'uint8','Signed', [ 0;],'Factor', [ 1;],'Offset', [ 0;],'Min', [ 0;],'Max', [ 0;],'Units', '','Comment', '','StartBit', [ 48;]),struct('Name', 'CMU1_Vcell_V16','Startbit', [ 0;],'SignalSize', [ 8;],'ByteOrder', 'BigEndian','ValueType', 'UNSIGNED','Class', 'uint8','Signed', [ 0;],'Factor', [ 1;],'Offset', [ 0;],'Min', [ 0;],'Max', [ 0;],'Units', '','Comment', '','StartBit', [ 56;])}}
      settings: SourceProductName=Raptor
  raptor_data_read : Raptor_lib/Data Storage/raptor_data_read  dataName='Rx_0x200C2A1_Cell_10_Volt'  dataShape=Scalar  idxSource=Input  idxRow=1  idxCol=1
      settings: SourceProductName=Raptor
  raptor_data_read1 : Raptor_lib/Data Storage/raptor_data_read  dataName='Rx_0x200C2A1_Cell_11_Volt'  dataShape=Scalar  idxSource=Input  idxRow=1  idxCol=1
      settings: SourceProductName=Raptor
  raptor_data_read2 : Raptor_lib/Data Storage/raptor_data_read  dataName='Rx_0x200C2A1_Cell_12_Volt'  dataShape=Scalar  idxSource=Input  idxRow=1  idxCol=1
      settings: SourceProductName=Raptor
  raptor_data_read3 : Raptor_lib/Data Storage/raptor_data_read  dataName='Rx_0x200C3A1_Cell_13_Volt'  dataShape=Scalar  idxSource=Input  idxRow=1  idxCol=1
      settings: SourceProductName=Raptor
  raptor_data_read4 : Raptor_lib/Data Storage/raptor_data_read  dataName='Rx_0x200C2A1_Cell_9_Volt'  dataShape=Scalar  idxSource=Input  idxRow=1  idxCol=1
      settings: SourceProductName=Raptor
  raptor_data_read5 : Raptor_lib/Data Storage/raptor_data_read  dataName='Rx_0x200C3A1_Cell_14_Volt'  dataShape=Scalar  idxSource=Input  idxRow=1  idxCol=1
      settings: SourceProductName=Raptor
  raptor_data_read6 : Raptor_lib/Data Storage/raptor_data_read  dataName='Rx_0x200C3A1_Cell_15_Volt'  dataShape=Scalar  idxSource=Input  idxRow=1  idxCol=1
      settings: SourceProductName=Raptor
  raptor_data_read7 : Raptor_lib/Data Storage/raptor_data_read  dataName='Rx_0x200C3A1_Cell_16_Volt'  dataShape=Scalar  idxSource=Input  idxRow=1  idxCol=1
      settings: SourceProductName=Raptor
  wires:
  Data Type Conversion4/1 -> raptor_can_txmsg/1
  Data Type Conversion8/1 -> raptor_can_txmsg/2
  Data Type Conversion7/1 -> raptor_can_txmsg/3
  Data Type Conversion6/1 -> raptor_can_txmsg/4
  Data Type Conversion1/1 -> raptor_can_txmsg/6
  Data Type Conversion2/1 -> raptor_can_txmsg/7
  Data Type Conversion3/1 -> raptor_can_txmsg/8
  raptor_data_read3/1 -> Fcn4/1
  Data Type Conversion5/1 -> raptor_can_txmsg/5
  raptor_data_read/1 -> Fcn1/1
  raptor_data_read1/1 -> Fcn2/1
  raptor_data_read2/1 -> Fcn3/1
  raptor_data_read4/1 -> Fcn/1
  raptor_data_read5/1 -> Fcn5/1
  raptor_data_read6/1 -> Fcn6/1
  raptor_data_read7/1 -> Fcn7/1
  Fcn/1 -> Data Type Conversion4/1
  Fcn1/1 -> Data Type Conversion8/1
  Fcn2/1 -> Data Type Conversion7/1
  Fcn3/1 -> Data Type Conversion6/1
  Fcn4/1 -> Data Type Conversion5/1
  Fcn5/1 -> Data Type Conversion1/1
  Fcn6/1 -> Data Type Conversion2/1
  Fcn7/1 -> Data Type Conversion3/1

== system EPT/Foreground_TimeBase_5ms/CAN/CAN1_exec/BCU vs RMDA-BMS/Remote DAG2-5E4 ==
  Trigger : TriggerPort  VariantControl=Variant  PortDimensions=1
  Data Type Conversion{1..8} (8 alike) : DataTypeConversion
  Fcn{1..8} (8 alike) : Fcn  Expr=(u(1)+40)/0.5
  raptor_can_txmsg : Raptor_lib/CAN/raptor_can_txmsg  canDefinition=struct('dbcFile', 'BCUvsRMDA_CMU.dbc','message', 'RemoteDAG_5E4','comment', '','signals', {{'CMU1_Tcell_T01','CMU1_Tcell_T02','CMU1_Tcell_T03','CMU1_Tcell_T04','CMU1_Tcell_T05','CMU1_Tcell_T06','CMU1_Tcell_T07','CMU1_Tcell_T08'}},'enabled', [ 1 1 1 1 1 1 1 1;],'canBus', '''CAN1''','messageID', [ 1508;],'idMask', [ 536870911;],'payloadMask', [],'payloadValue', [],'period', [ 0;],'mailbox', '','queueSize', [ 1;],'label', [ 0;],'ver', [ 2;],'showID', [ 0;],'showRaw', [ 0;],'fill', [ 0;],'editID', [ 0;],'signalOrder', [ 1;])  canBus='CAN1'  queueSize=1  payloadMask=[]  payloadValue=[]  period=0  showID=0  label=0  idMask=hex2dec('1FFFFFFF')  fill=0  id=1508  showRaw=0  signalOrder=1  signalInfo={{struct('Name', 'CMU1_Tcell_T01','Startbit', [ 0;],'SignalSize', [ 8;],'ByteOrder', 'BigEndian','ValueType', 'UNSIGNED','Class', 'uint8','Signed', [ 0;],'Factor', [ 1;],'Offset', [ 0;],'Min', [ 0;],'Max', [ 0;],'Units', '','Comment', '','StartBit', [ 0;]),struct('Name', 'CMU1_Tcell_T02','Startbit', [ 0;],'SignalSize', [ 8;],'ByteOrder', 'BigEndian','ValueType', 'UNSIGNED','Class', 'uint8','Signed', [ 0;],'Factor', [ 1;],'Offset', [ 0;],'Min', [ 0;],'Max', [ 0;],'Units', '','Comment', '','StartBit', [ 8;]),struct('Name', 'CMU1_Tcell_T03','Startbit', [ 0;],'SignalSize', [ 8;],'ByteOrder', 'BigEndian','ValueType', 'UNSIGNED','Class', 'uint8','Signed', [ 0;],'Factor', [ 1;],'Offset', [ 0;],'Min', [ 0;],'Max', [ 0;],'Units', '','Comment', '','StartBit', [ 16;]),struct('Name', 'CMU1_Tcell_T04','Startbit', [ 0;],'SignalSize', [ 8;],'ByteOrder', 'BigEndian','ValueType', 'UNSIGNED','Class', 'uint8','Signed', [ 0;],'Factor', [ 1;],'Offset', [ 0;],'Min', [ 0;],'Max', [ 0;],'Units', '','Comment', '','StartBit', [ 24;]),struct('Name', 'CMU1_Tcell_T05','Startbit', [ 0;],'SignalSize', [ 8;],'ByteOrder', 'BigEndian','ValueType', 'UNSIGNED','Class', 'uint8','Signed', [ 0;],'Factor', [ 1;],'Offset', [ 0;],'Min', [ 0;],'Max', [ 0;],'Units', '','Comment', '','StartBit', [ 32;]),struct('Name', 'CMU1_Tcell_T06','Startbit', [ 0;],'SignalSize', [ 8;],'ByteOrder', 'BigEndian','ValueType', 'UNSIGNED','Class', 'uint8','Signed', [ 0;],'Factor', [ 1;],'Offset', [ 0;],'Min', [ 0;],'Max', [ 0;],'Units', '','Comment', '','StartBit', [ 40;]),struct('Name', 'CMU1_Tcell_T07','Startbit', [ 0;],'SignalSize', [ 8;],'ByteOrder', 'BigEndian','ValueType', 'UNSIGNED','Class', 'uint8','Signed', [ 0;],'Factor', [ 1;],'Offset', [ 0;],'Min', [ 0;],'Max', [ 0;],'Units', '','Comment', '','StartBit', [ 48;]),struct('Name', 'CMU1_Tcell_T08','Startbit', [ 0;],'SignalSize', [ 8;],'ByteOrder', 'BigEndian','ValueType', 'UNSIGNED','Class', 'uint8','Signed', [ 0;],'Factor', [ 1;],'Offset', [ 0;],'Min', [ 0;],'Max', [ 0;],'Units', '','Comment', '','StartBit', [ 56;])}}
      settings: SourceProductName=Raptor
  raptor_data_read : Raptor_lib/Data Storage/raptor_data_read  dataName='Rx_0x200C4A1_Cell_1_Temp'  dataShape=Scalar  idxSource=Input  idxRow=1  idxCol=1
      settings: SourceProductName=Raptor
  raptor_data_read1 : Raptor_lib/Data Storage/raptor_data_read  dataName='Rx_0x200C4A1_Cell_2_Temp'  dataShape=Scalar  idxSource=Input  idxRow=1  idxCol=1
      settings: SourceProductName=Raptor
  raptor_data_read2 : Raptor_lib/Data Storage/raptor_data_read  dataName='Rx_0x200C4A1_Cell_3_Temp'  dataShape=Scalar  idxSource=Input  idxRow=1  idxCol=1
      settings: SourceProductName=Raptor
  raptor_data_read3 : Raptor_lib/Data Storage/raptor_data_read  dataName='Rx_0x200C4A1_Cell_4_Temp'  dataShape=Scalar  idxSource=Input  idxRow=1  idxCol=1
      settings: SourceProductName=Raptor
  raptor_data_read4 : Raptor_lib/Data Storage/raptor_data_read  dataName='Rx_0x200C5A1_Cell_5_Temp'  dataShape=Scalar  idxSource=Input  idxRow=1  idxCol=1
      settings: SourceProductName=Raptor
  raptor_data_read5 : Raptor_lib/Data Storage/raptor_data_read  dataName='Rx_0x200C5A1_Cell_6_Temp'  dataShape=Scalar  idxSource=Input  idxRow=1  idxCol=1
      settings: SourceProductName=Raptor
  raptor_data_read6 : Raptor_lib/Data Storage/raptor_data_read  dataName='Rx_0x200C5A1_Cell_7_Temp'  dataShape=Scalar  idxSource=Input  idxRow=1  idxCol=1
      settings: SourceProductName=Raptor
  raptor_data_read7 : Raptor_lib/Data Storage/raptor_data_read  dataName='Rx_0x200C5A1_Cell_8_Temp'  dataShape=Scalar  idxSource=Input  idxRow=1  idxCol=1
      settings: SourceProductName=Raptor
  wires:
  raptor_data_read3/1 -> Fcn4/1
  raptor_data_read2/1 -> Fcn3/1
  raptor_data_read1/1 -> Fcn1/1
  raptor_data_read/1 -> Fcn2/1
  raptor_data_read4/1 -> Fcn5/1
  raptor_data_read5/1 -> Fcn6/1
  raptor_data_read6/1 -> Fcn7/1
  raptor_data_read7/1 -> Fcn8/1
  Fcn2/1 -> Data Type Conversion3/1
  Fcn1/1 -> Data Type Conversion1/1
  Fcn3/1 -> Data Type Conversion2/1
  Fcn4/1 -> Data Type Conversion4/1
  Fcn5/1 -> Data Type Conversion5/1
  Fcn6/1 -> Data Type Conversion6/1
  Fcn7/1 -> Data Type Conversion7/1
  Fcn8/1 -> Data Type Conversion8/1
  Data Type Conversion3/1 -> raptor_can_txmsg/1
  Data Type Conversion1/1 -> raptor_can_txmsg/2
  Data Type Conversion2/1 -> raptor_can_txmsg/3
  Data Type Conversion4/1 -> raptor_can_txmsg/4
  Data Type Conversion5/1 -> raptor_can_txmsg/5
  Data Type Conversion6/1 -> raptor_can_txmsg/6
  Data Type Conversion7/1 -> raptor_can_txmsg/7
  Data Type Conversion8/1 -> raptor_can_txmsg/8

== system EPT/Foreground_TimeBase_5ms/CAN/CAN1_exec/BCU vs RMDA-BMS/Remote DAG2-5E5 ==
  Trigger : TriggerPort  VariantControl=Variant  PortDimensions=1
  Data Type Conversion{1..8} (8 alike) : DataTypeConversion
  Fcn{1..8} (8 alike) : Fcn  Expr=(u(1)+40)/0.5
  raptor_can_txmsg : Raptor_lib/CAN/raptor_can_txmsg  canDefinition=struct('dbcFile', 'BCUvsRMDA_CMU.dbc','message', 'RemoteDAG_5E5','comment', '','signals', {{'CMU1_Tcell_T09','CMU1_Tcell_T10','CMU1_Tcell_T11','CMU1_Tcell_T12','CMU1_Tcell_T13','CMU1_Tcell_T14','CMU1_Tcell_T15','CMU1_Tcell_T16'}},'enabled', [ 1 1 1 1 1 1 1 1;],'canBus', '''CAN1''','messageID', [ 1509;],'idMask', [ 536870911;],'payloadMask', [],'payloadValue', [],'period', [ 0;],'mailbox', '','queueSize', [ 1;],'label', [ 0;],'ver', [ 2;],'showID', [ 0;],'showRaw', [ 0;],'fill', [ 0;],'editID', [ 0;],'signalOrder', [ 1;])  canBus='CAN1'  queueSize=1  payloadMask=[]  payloadValue=[]  period=0  showID=0  label=0  idMask=hex2dec('1FFFFFFF')  fill=0  id=1509  showRaw=0  signalOrder=1  signalInfo={{struct('Name', 'CMU1_Tcell_T09','Startbit', [ 0;],'SignalSize', [ 8;],'ByteOrder', 'BigEndian','ValueType', 'UNSIGNED','Class', 'uint8','Signed', [ 0;],'Factor', [ 1;],'Offset', [ 0;],'Min', [ 0;],'Max', [ 0;],'Units', '','Comment', '','StartBit', [ 0;]),struct('Name', 'CMU1_Tcell_T10','Startbit', [ 0;],'SignalSize', [ 8;],'ByteOrder', 'BigEndian','ValueType', 'UNSIGNED','Class', 'uint8','Signed', [ 0;],'Factor', [ 1;],'Offset', [ 0;],'Min', [ 0;],'Max', [ 0;],'Units', '','Comment', '','StartBit', [ 8;]),struct('Name', 'CMU1_Tcell_T11','Startbit', [ 0;],'SignalSize', [ 8;],'ByteOrder', 'BigEndian','ValueType', 'UNSIGNED','Class', 'uint8','Signed', [ 0;],'Factor', [ 1;],'Offset', [ 0;],'Min', [ 0;],'Max', [ 0;],'Units', '','Comment', '','StartBit', [ 16;]),struct('Name', 'CMU1_Tcell_T12','Startbit', [ 0;],'SignalSize', [ 8;],'ByteOrder', 'BigEndian','ValueType', 'UNSIGNED','Class', 'uint8','Signed', [ 0;],'Factor', [ 1;],'Offset', [ 0;],'Min', [ 0;],'Max', [ 0;],'Units', '','Comment', '','StartBit', [ 24;]),struct('Name', 'CMU1_Tcell_T13','Startbit', [ 0;],'SignalSize', [ 8;],'ByteOrder', 'BigEndian','ValueType', 'UNSIGNED','Class', 'uint8','Signed', [ 0;],'Factor', [ 1;],'Offset', [ 0;],'Min', [ 0;],'Max', [ 0;],'Units', '','Comment', '','StartBit', [ 32;]),struct('Name', 'CMU1_Tcell_T14','Startbit', [ 0;],'SignalSize', [ 8;],'ByteOrder', 'BigEndian','ValueType', 'UNSIGNED','Class', 'uint8','Signed', [ 0;],'Factor', [ 1;],'Offset', [ 0;],'Min', [ 0;],'Max', [ 0;],'Units', '','Comment', '','StartBit', [ 40;]),struct('Name', 'CMU1_Tcell_T15','Startbit', [ 0;],'SignalSize', [ 8;],'ByteOrder', 'BigEndian','ValueType', 'UNSIGNED','Class', 'uint8','Signed', [ 0;],'Factor', [ 1;],'Offset', [ 0;],'Min', [ 0;],'Max', [ 0;],'Units', '','Comment', '','StartBit', [ 48;]),struct('Name', 'CMU1_Tcell_T16','Startbit', [ 0;],'SignalSize', [ 8;],'ByteOrder', 'BigEndian','ValueType', 'UNSIGNED','Class', 'uint8','Signed', [ 0;],'Factor', [ 1;],'Offset', [ 0;],'Min', [ 0;],'Max', [ 0;],'Units', '','Comment', '','StartBit', [ 56;])}}
      settings: SourceProductName=Raptor
  raptor_data_read : Raptor_lib/Data Storage/raptor_data_read  dataName='Rx_0x200C6A1_Cell_9_Temp'  dataShape=Scalar  idxSource=Input  idxRow=1  idxCol=1
      settings: SourceProductName=Raptor
  raptor_data_read1 : Raptor_lib/Data Storage/raptor_data_read  dataName='Rx_0x200C6A1_Cell_10_Temp'  dataShape=Scalar  idxSource=Input  idxRow=1  idxCol=1
      settings: SourceProductName=Raptor
  raptor_data_read2 : Raptor_lib/Data Storage/raptor_data_read  dataName='Rx_0x200C6A1_Cell_11_Temp'  dataShape=Scalar  idxSource=Input  idxRow=1  idxCol=1
      settings: SourceProductName=Raptor
  raptor_data_read3 : Raptor_lib/Data Storage/raptor_data_read  dataName='Rx_0x200C6A1_Cell_12_Temp'  dataShape=Scalar  idxSource=Input  idxRow=1  idxCol=1
      settings: SourceProductName=Raptor
  raptor_data_read4 : Raptor_lib/Data Storage/raptor_data_read  dataName='Rx_0x200C7A1_Cell_13_Temp'  dataShape=Scalar  idxSource=Input  idxRow=1  idxCol=1
      settings: SourceProductName=Raptor
  raptor_data_read5 : Raptor_lib/Data Storage/raptor_data_read  dataName='Rx_0x200C7A1_Cell_14_Temp'  dataShape=Scalar  idxSource=Input  idxRow=1  idxCol=1
      settings: SourceProductName=Raptor
  raptor_data_read6 : Raptor_lib/Data Storage/raptor_data_read  dataName='Rx_0x200C7A1_Cell_15_Temp'  dataShape=Scalar  idxSource=Input  idxRow=1  idxCol=1
      settings: SourceProductName=Raptor
  raptor_data_read7 : Raptor_lib/Data Storage/raptor_data_read  dataName='Rx_0x200C7A1_Cell_16_Temp'  dataShape=Scalar  idxSource=Input  idxRow=1  idxCol=1
      settings: SourceProductName=Raptor
  wires:
  Data Type Conversion8/1 -> raptor_can_txmsg/8
  Data Type Conversion7/1 -> raptor_can_txmsg/7
  Data Type Conversion4/1 -> raptor_can_txmsg/4
  raptor_data_read/1 -> Fcn2/1
  Data Type Conversion2/1 -> raptor_can_txmsg/3
  Data Type Conversion6/1 -> raptor_can_txmsg/6
  raptor_data_read4/1 -> Fcn5/1
  raptor_data_read7/1 -> Fcn8/1
  raptor_data_read5/1 -> Fcn6/1
  raptor_data_read6/1 -> Fcn7/1
  raptor_data_read1/1 -> Fcn1/1
  raptor_data_read3/1 -> Fcn4/1
  Data Type Conversion1/1 -> raptor_can_txmsg/2
  raptor_data_read2/1 -> Fcn3/1
  Fcn2/1 -> Data Type Conversion3/1
  Fcn8/1 -> Data Type Conversion8/1
  Fcn1/1 -> Data Type Conversion1/1
  Fcn6/1 -> Data Type Conversion6/1
  Fcn4/1 -> Data Type Conversion4/1
  Data Type Conversion3/1 -> raptor_can_txmsg/1
  Data Type Conversion5/1 -> raptor_can_txmsg/5
  Fcn5/1 -> Data Type Conversion5/1
  Fcn7/1 -> Data Type Conversion7/1
  Fcn3/1 -> Data Type Conversion2/1
